simulink library "fec"  (Simulink 8.1)
settings: Solver=ode1  StartTime=0.0  StopTime=Inf  FixedStep=0.001  RelTol=1e-3
PostLoadFcn:
  | , if any(exist('dsrtsu_mdlpostloadfcn', 'file') == [2, 3, 6]), try dsrtsu_mdlpostloadfcn('Execute', bdroot); catch fprintf('Error in PostLoadFcn (dsrtsu_mdlpostloadfcn) for model "%s":\n %s\n', bdroot, lasterr); end, end,
undefined symbols (not defined in the file): ENUM_KEYSWITCH_ON, ENUM_SENSORSTATE_NORMAL
settings Model: DSRTSU_INTERNAL_RTI_VER=450  DSRTSU_INTERNAL_RTI_TYPE=rti1401  RTICANMMDATA=struct('GeneralSetupData',struct('modelroot',['D:\Soichi\SVNDATA\haitec_adas\Model Based Design\HAITEC\AdasDragon\software\sw_development\arch\app\jud\jcw\fec'],'generalsettings',struct('filesettings',struct('destfolder',struct('Name','RTICANMM_FILES','Check',1),'buildfolder',struct('Name','.','Check',1),'AbsDestfolder',struct('Name',['D:\Soichi\SVNDATA\haitec_adas\Model Based Design\HAITEC\AdasDragon\software\sw_development\arch\app\jud\jcw\fec\RTICANMM_FILES']),'AbsBuildfolder',struct('Name',['D:\Soichi\SVNDATA\haitec_adas\Model Based Design\HAITEC\AdasDragon\software\sw_development\arch\app\jud\jcw\fec']))),'options',struct('addpaths',1,'rmpaths',1,'addtrcexclusion',logical(1),'cannavigator',struct('checkmonitoring',0),'show_usrtrc',0,'use_usrtrc',0),'advanced',struct('options',[1 1 1 1 1 1 1 1 1 1 1 1 1 1 1 1 1 1 1 1 1 1 1 1 1 1 1 1 1 1 1 1 1 1 1 1 1 1 1 1 1 1 1 1 1 1 1 1 1 1 1 1 1 1 1 1 1 1 1 1 1 1 1 1 1 1 1 1 1 1 1 1 1 1 1 1 1 1 1 1 1 1 1 1 1 1 1 1 1 1 1 1 1 1 1 1 1 1 1 1]),'MPSetup',{{}},'modelname','fec','block','fec'))  DSRTSU_INTERNAL_RTIFPGA=40  Creator=AT015411  LastModifiedBy=idiada

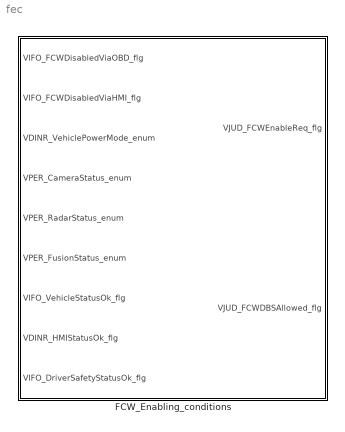
== system fec ==
  FCW_Enabling_conditions : Subsystem

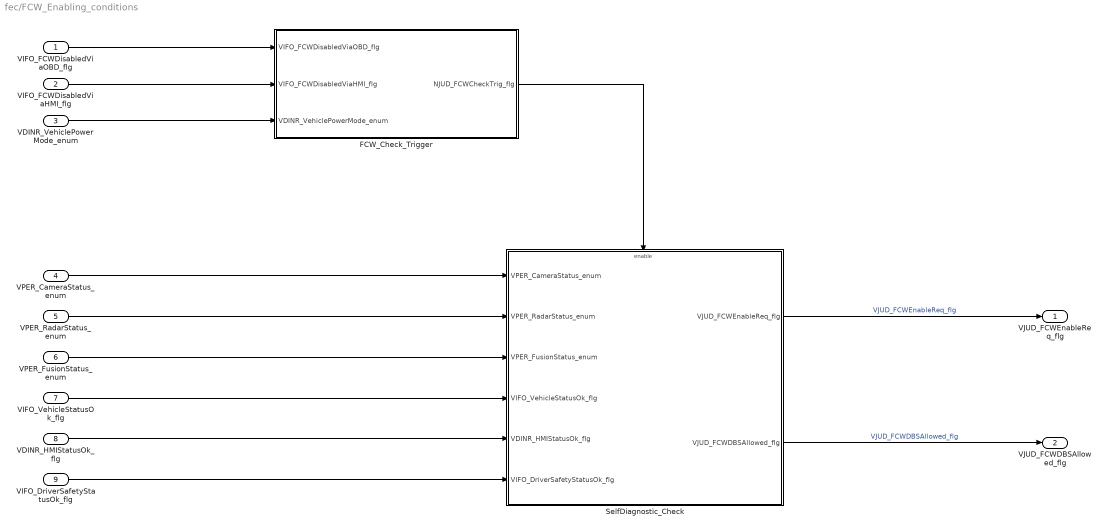
== system fec/FCW_Enabling_conditions ==
  VIFO_FCWDisabledViaOBD_flg : Inport
  VIFO_FCWDisabledViaHMI_flg : Inport  Port=2
  VDINR_VehiclePowerMode_enum : Inport  Port=3
  VPER_CameraStatus_enum : Inport  Port=4
  VPER_RadarStatus_enum : Inport  Port=5
  VPER_FusionStatus_enum : Inport  Port=6
  VIFO_VehicleStatusOk_flg : Inport  Port=7
  VDINR_HMIStatusOk_flg : Inport  Port=8
  VIFO_DriverSafetyStatusOk_flg : Inport  Port=9
  FCW_Check_Trigger : Subsystem
  SelfDiagnostic_Check : Subsystem
  VJUD_FCWEnableReq_flg : Outport
  VJUD_FCWDBSAllowed_flg : Outport  Port=2
  wires:
  VPER_CameraStatus_enum/1 -> SelfDiagnostic_Check/1(VPER_CameraStatus_enum)
  VPER_RadarStatus_enum/1 -> SelfDiagnostic_Check/2(VPER_RadarStatus_enum)
  VPER_FusionStatus_enum/1 -> SelfDiagnostic_Check/3(VPER_FusionStatus_enum)
  VIFO_VehicleStatusOk_flg/1 -> SelfDiagnostic_Check/4(VIFO_VehicleStatusOk_flg)
  VDINR_HMIStatusOk_flg/1 -> SelfDiagnostic_Check/5(VDINR_HMIStatusOk_flg)
  VIFO_DriverSafetyStatusOk_flg/1 -> SelfDiagnostic_Check/6(VIFO_DriverSafetyStatusOk_flg)
  SelfDiagnostic_Check/1(VJUD_FCWEnableReq_flg) -> VJUD_FCWEnableReq_flg/1  "VJUD_FCWEnableReq_flg"
  SelfDiagnostic_Check/2(VJUD_FCWDBSAllowed_flg) -> VJUD_FCWDBSAllowed_flg/1  "VJUD_FCWDBSAllowed_flg"
  VIFO_FCWDisabledViaOBD_flg/1 -> FCW_Check_Trigger/1(VIFO_FCWDisabledViaOBD_flg)
  VIFO_FCWDisabledViaHMI_flg/1 -> FCW_Check_Trigger/2(VIFO_FCWDisabledViaHMI_flg)
  VDINR_VehiclePowerMode_enum/1 -> FCW_Check_Trigger/3(VDINR_VehiclePowerMode_enum)
  FCW_Check_Trigger/1(NJUD_FCWCheckTrig_flg) -> SelfDiagnostic_Check/Enable

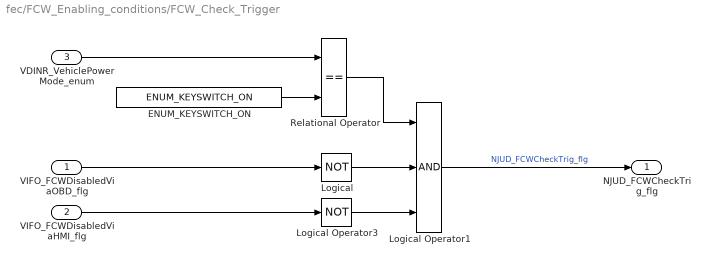
== system fec/FCW_Enabling_conditions/FCW_Check_Trigger ==
  VIFO_FCWDisabledViaOBD_flg : Inport
  VIFO_FCWDisabledViaHMI_flg : Inport  Port=2
  VDINR_VehiclePowerMode_enum : Inport  Port=3
  ENUM_KEYSWITCH_ON : Constant  Value=ENUM_KEYSWITCH_ON  OutDataTypeStr=uint8
  Logical : Logic  Operator=NOT  Inputs=3  AllPortsSameDT=off  OutDataTypeStr=boolean
  Logical Operator1 : Logic  Inputs=3  AllPortsSameDT=off  OutDataTypeStr=boolean
  Logical Operator3 : Logic  Operator=NOT  Inputs=3  AllPortsSameDT=off  OutDataTypeStr=boolean
  Relational Operator : RelationalOperator  Operator===  OutDataTypeStr=boolean
  NJUD_FCWCheckTrig_flg : Outport
  wires:
  ENUM_KEYSWITCH_ON/1 -> Relational Operator/2
  VDINR_VehiclePowerMode_enum/1 -> Relational Operator/1
  Logical/1 -> Logical Operator1/2
  VIFO_FCWDisabledViaOBD_flg/1 -> Logical/1
  Logical Operator3/1 -> Logical Operator1/3
  Relational Operator/1 -> Logical Operator1/1
  Logical Operator1/1 -> NJUD_FCWCheckTrig_flg/1  "NJUD_FCWCheckTrig_flg"
  VIFO_FCWDisabledViaHMI_flg/1 -> Logical Operator3/1

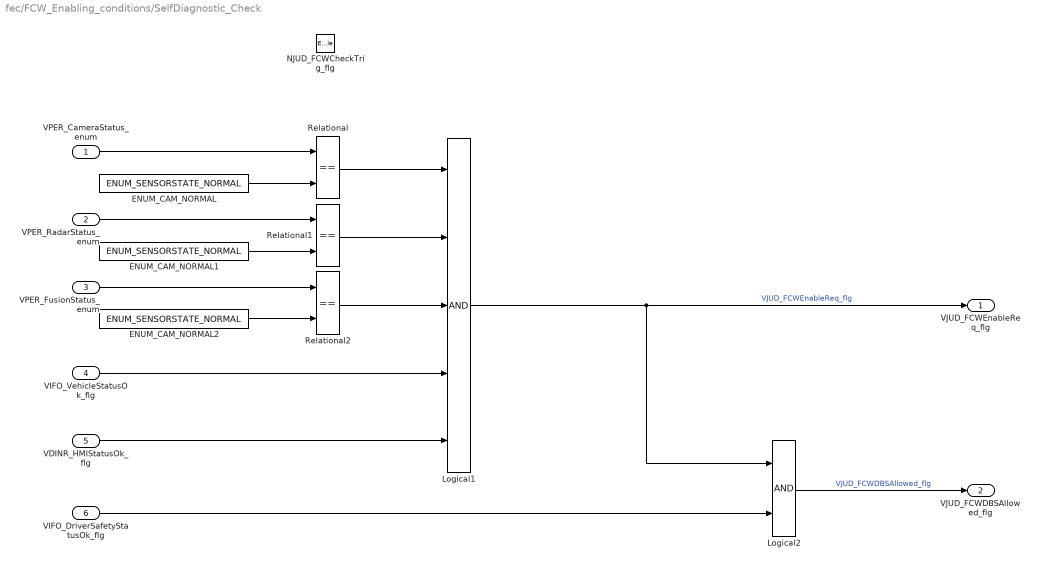
== system fec/FCW_Enabling_conditions/SelfDiagnostic_Check ==
  VPER_CameraStatus_enum : Inport
  VPER_RadarStatus_enum : Inport  Port=2
  VPER_FusionStatus_enum : Inport  Port=3
  VIFO_VehicleStatusOk_flg : Inport  Port=4
  VDINR_HMIStatusOk_flg : Inport  Port=5
  VIFO_DriverSafetyStatusOk_flg : Inport  Port=6
  NJUD_FCWCheckTrig_flg : EnablePort  StatesWhenEnabling=reset
      settings: AttributesFormatString=State =%<StatesWhenEnabling>
  ENUM_CAM_NORMAL : Constant  Value=ENUM_SENSORSTATE_NORMAL  OutDataTypeStr=uint8
  ENUM_CAM_NORMAL1 : Constant  Value=ENUM_SENSORSTATE_NORMAL  OutDataTypeStr=uint8
  ENUM_CAM_NORMAL2 : Constant  Value=ENUM_SENSORSTATE_NORMAL  OutDataTypeStr=uint8
  Logical1 : Logic  Inputs=5  AllPortsSameDT=off  OutDataTypeStr=boolean
  Logical2 : Logic  AllPortsSameDT=off  OutDataTypeStr=boolean
  Relational : RelationalOperator  Operator===  OutDataTypeStr=boolean
  Relational1 : RelationalOperator  Operator===  OutDataTypeStr=boolean
  Relational2 : RelationalOperator  Operator===  OutDataTypeStr=boolean
  VJUD_FCWEnableReq_flg : Outport  OutputWhenDisabled=reset  InitialOutput=0
  VJUD_FCWDBSAllowed_flg : Outport  Port=2  OutputWhenDisabled=reset  InitialOutput=0
  wires:
  VPER_CameraStatus_enum/1 -> Relational/1
  ENUM_CAM_NORMAL/1 -> Relational/2
  VDINR_HMIStatusOk_flg/1 -> Logical1/5
  Relational/1 -> Logical1/1
  Relational1/1 -> Logical1/2
  VIFO_VehicleStatusOk_flg/1 -> Logical1/4
  Logical1/1 -> Logical2/1, VJUD_FCWEnableReq_flg/1  "VJUD_FCWEnableReq_flg"
  VIFO_DriverSafetyStatusOk_flg/1 -> Logical2/2
  Logical2/1 -> VJUD_FCWDBSAllowed_flg/1  "VJUD_FCWDBSAllowed_flg"
  VPER_RadarStatus_enum/1 -> Relational1/1
  ENUM_CAM_NORMAL1/1 -> Relational1/2
  Relational2/1 -> Logical1/3
  VPER_FusionStatus_enum/1 -> Relational2/1
  ENUM_CAM_NORMAL2/1 -> Relational2/2
